simulink model "Diffsion"  (R2022b)
settings: Solver=FixedStepDiscrete  StartTime=0.0  StopTime=10.0  RelTol=1e-3
libraries: simulink x1
settings Model: Creator=yuzehong  LastModifiedBy=yuzehong
settings SolverCC: AlgebraicLoopSolver=TrustRegion
settings OptimizationCC: DefaultParameterBehavior=Inlined  EnhancedBackFolding=on  PassReuseOutputArgsAs=Individual arguments  OptimizeBlockOrder=speed  DifferentSizesBufferReuse=on  EfficientTunableParamExpr=on
settings DebuggingCC: ParameterTunabilityLossMsg=error
settings SFSimCC: MATLABDynamicMemAlloc=off
settings RTWCC: Description=Embedded Coder  SystemTargetFile=ert.tlc  GenCodeOnly=on  TemplateMakefile=ert_default_tmf
settings CodeAppCC: GenerateComments=off  IgnoreCustomStorageClasses=off  OperatorAnnotations=on  SimulinkDataObjDesc=on  SFDataObjDesc=on  SimulinkBlockComments=off
settings ERTTargetCC: TargetLangStandard=C99 (ISO)  GenerateSampleERTMain=on  CodeInterfacePackaging=Reusable function  InlinedParameterPlacement=NonHierarchical  ERTCustomFileTemplate=example_file_process.tlc

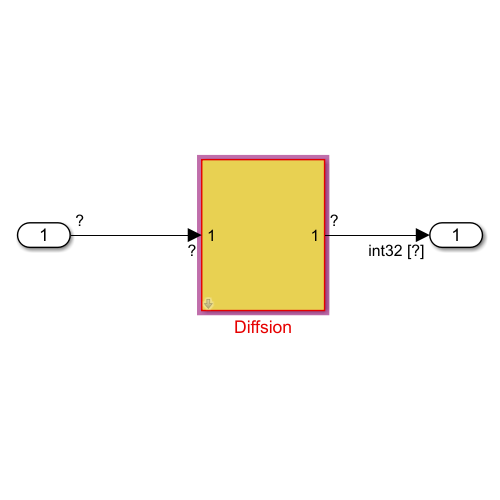
[thumbnail: Simulink's stored preview of the top-level diagram]
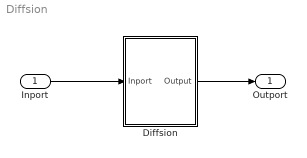
== system Diffsion ==
  Inport : Inport
  Diffsion : Subsystem  mask{length=32}
  Outport : Outport  OutDataTypeStr=int32
  wires:
  Diffsion/1(Output) -> Outport/1
  Inport/1 -> Diffsion/1(Inport)

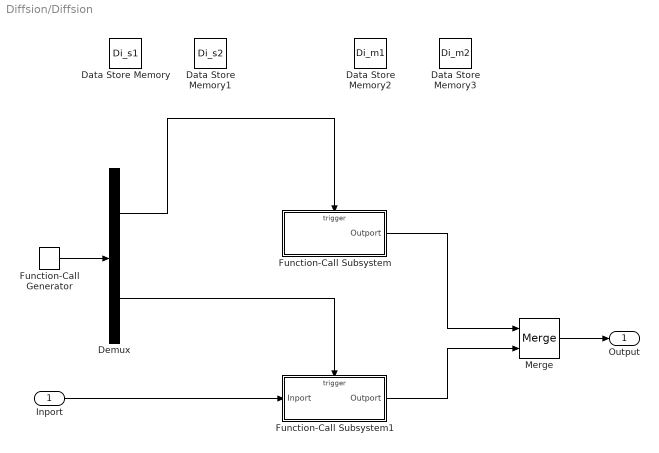
== system Diffsion/Diffsion ==
  Inport : Inport
  Data Store Memory : DataStoreMemory  DataStoreName=Di_s1  WriteAfterWriteMsg=warning  ShowAdditionalParam=off  OutDataTypeStr=int32  Dimensions=length
  Data Store Memory1 : DataStoreMemory  DataStoreName=Di_s2  WriteAfterWriteMsg=warning  ShowAdditionalParam=off  OutDataTypeStr=int32  Dimensions=length
  Data Store Memory2 : DataStoreMemory  DataStoreName=Di_m1  WriteAfterWriteMsg=warning  ShowAdditionalParam=off  OutDataTypeStr=int32  Dimensions=length
  Data Store Memory3 : DataStoreMemory  DataStoreName=Di_m2  WriteAfterWriteMsg=warning  ShowAdditionalParam=off  OutDataTypeStr=int32  Dimensions=length
  Demux : Demux  Outputs=2
  Function-Call Generator : simulink/Ports & Subsystems/Function-Call Generator  sample_time=1  numberOfIterations=1  DisallowWideOutput=off
  Function-Call Subsystem : Subsystem  TreatAsAtomicUnit=on
  Function-Call Subsystem1 : Subsystem  TreatAsAtomicUnit=on
  Merge : Merge
  Output : Outport
  wires:
  Function-Call Generator/1 -> Demux/1
  Demux/1 -> Function-Call Subsystem/Trigger
  Demux/2 -> Function-Call Subsystem1/Trigger
  Inport/1 -> Function-Call Subsystem1/1(Inport)
  Function-Call Subsystem/1(Outport) -> Merge/1
  Function-Call Subsystem1/1(Outport) -> Merge/2
  Merge/1 -> Output/1

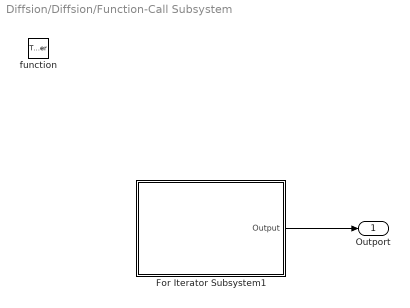
== system Diffsion/Diffsion/Function-Call Subsystem ==
  function : TriggerPort  TriggerType=function-call  VariantControl=(inherit)
  For Iterator Subsystem1 : Subsystem  TreatAsAtomicUnit=on
  Outport : Outport  OutDataTypeStr=int32
  wires:
  For Iterator Subsystem1/1(Output) -> Outport/1

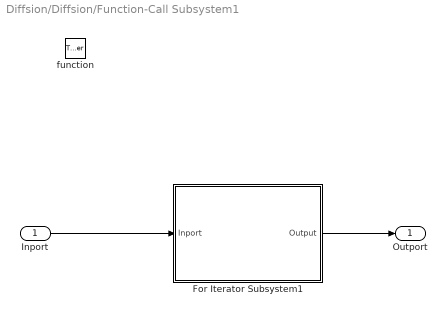
== system Diffsion/Diffsion/Function-Call Subsystem1 ==
  Inport : Inport  OutDataTypeStr=int32
  function : TriggerPort  TriggerType=function-call  VariantControl=(inherit)
  For Iterator Subsystem1 : Subsystem  TreatAsAtomicUnit=on
  Outport : Outport  OutDataTypeStr=int32
  wires:
  For Iterator Subsystem1/1(Output) -> Outport/1
  Inport/1 -> For Iterator Subsystem1/1(Inport)

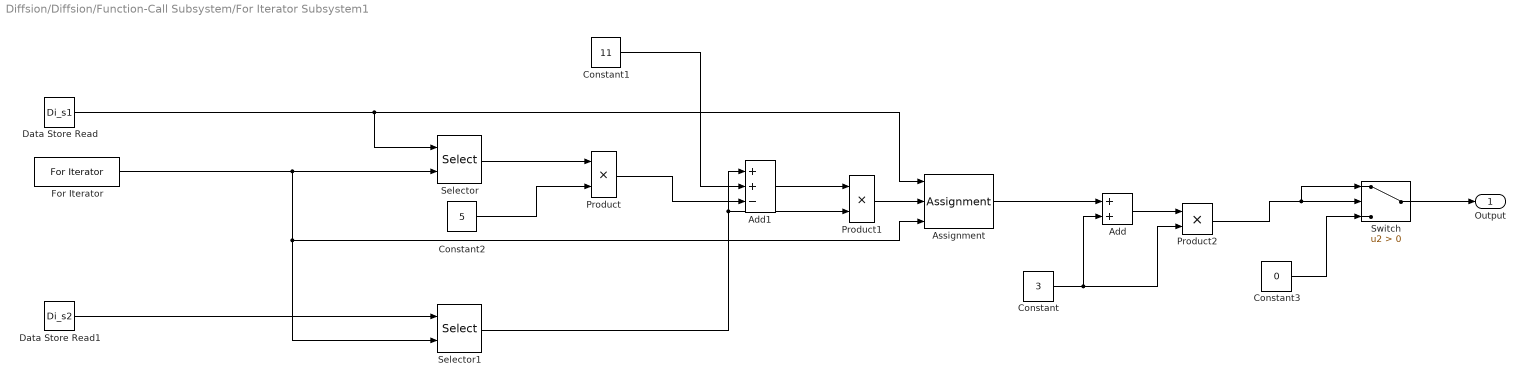
== system Diffsion/Diffsion/Function-Call Subsystem/For Iterator Subsystem1 ==
  Add : Sum  AccumDataTypeStr=int32
  Add1 : Sum  Inputs=++-  AccumDataTypeStr=int32  OutDataTypeStr=int32
  Assignment : Assignment  IndexMode=Zero-based  DiagnosticForDimensions=Warning  IndexOptions=Index vector (port)  Indices=1  OutputSizes=1
  Constant : Constant  Value=3  OutDataTypeStr=int32
  Constant1 : Constant  Value=11  OutDataTypeStr=int32
  Constant2 : Constant  Value=5  OutDataTypeStr=int32
  Constant3 : Constant  Value=0  OutDataTypeStr=int32
  Data Store Read : DataStoreRead  DataStoreName=Di_s1  IndexOptions=Index vector (dialog)  Indices=1  OutputSizes=1
  Data Store Read1 : DataStoreRead  DataStoreName=Di_s2  IndexOptions=Index vector (dialog)  Indices=1  OutputSizes=1
  For Iterator : ForIterator  IterationLimit=length  IndexMode=Zero-based
  Product : Product  OutDataTypeStr=int32
  Product1 : Product  OutDataTypeStr=int32
  Product2 : Product  OutDataTypeStr=int32
  Selector : Selector  IndexMode=Zero-based  InputPortWidth=length  IndexOptions=Index vector (port)  Indices=[1 3]  OutputSizes=1
  Selector1 : Selector  IndexMode=Zero-based  InputPortWidth=length  IndexOptions=Index vector (port)  Indices=[1 3]  OutputSizes=1
  Switch : Switch  Criteria=u2 > Threshold  SaturateOnIntegerOverflow=off  InputSameDT=off
  Output : Outport  OutDataTypeStr=int32
  wires:
  Data Store Read/1 -> Selector/1, Assignment/1
  For Iterator/1 -> Selector1/2, Assignment/3, Selector/2
  Constant2/1 -> Product/2
  Selector/1 -> Product/1
  Product/1 -> Add1/3
  Add1/1 -> Product1/1
  Product1/1 -> Assignment/2
  Constant1/1 -> Add1/2
  Data Store Read1/1 -> Selector1/1
  Selector1/1 -> Add1/1, Product1/2
  Switch/1 -> Output/1
  Constant3/1 -> Switch/3
  Assignment/1 -> Add/1
  Constant/1 -> Product2/2, Add/2
  Add/1 -> Product2/1
  Product2/1 -> Switch/1, Switch/2

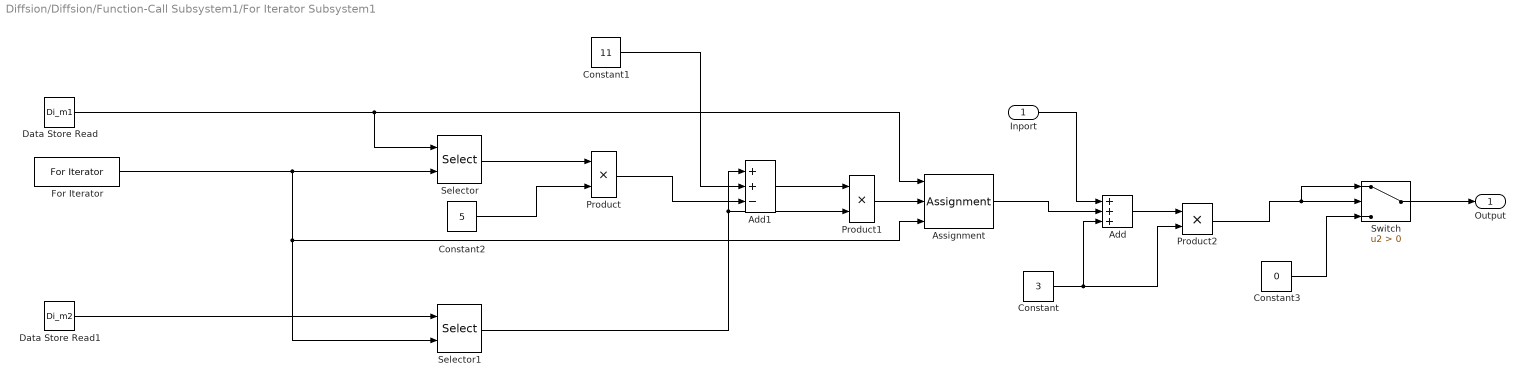
== system Diffsion/Diffsion/Function-Call Subsystem1/For Iterator Subsystem1 ==
  Inport : Inport  OutDataTypeStr=int32
  Add : Sum  Inputs=+++  AccumDataTypeStr=int32  OutDataTypeStr=int32
  Add1 : Sum  Inputs=++-  AccumDataTypeStr=int32  OutDataTypeStr=int32
  Assignment : Assignment  IndexMode=Zero-based  DiagnosticForDimensions=Warning  IndexOptions=Index vector (port)  Indices=1  OutputSizes=1
  Constant : Constant  Value=3  OutDataTypeStr=int32
  Constant1 : Constant  Value=11  OutDataTypeStr=int32
  Constant2 : Constant  Value=5  OutDataTypeStr=int32
  Constant3 : Constant  Value=0  OutDataTypeStr=int32
  Data Store Read : DataStoreRead  DataStoreName=Di_m1  IndexOptions=Index vector (dialog)  Indices=1  OutputSizes=1
  Data Store Read1 : DataStoreRead  DataStoreName=Di_m2  IndexOptions=Index vector (dialog)  Indices=1  OutputSizes=1
  For Iterator : ForIterator  IterationLimit=length  IndexMode=Zero-based
  Product : Product  OutDataTypeStr=int32
  Product1 : Product  OutDataTypeStr=int32
  Product2 : Product  OutDataTypeStr=int32
  Selector : Selector  IndexMode=Zero-based  InputPortWidth=length  IndexOptions=Index vector (port)  Indices=[1 3]  OutputSizes=1
  Selector1 : Selector  IndexMode=Zero-based  InputPortWidth=length  IndexOptions=Index vector (port)  Indices=[1 3]  OutputSizes=1
  Switch : Switch  Criteria=u2 > Threshold  SaturateOnIntegerOverflow=off  InputSameDT=off
  Output : Outport  OutDataTypeStr=int32
  wires:
  Data Store Read/1 -> Selector/1, Assignment/1
  For Iterator/1 -> Selector1/2, Assignment/3, Selector/2
  Constant2/1 -> Product/2
  Selector/1 -> Product/1
  Product/1 -> Add1/3
  Add1/1 -> Product1/1
  Product1/1 -> Assignment/2
  Constant1/1 -> Add1/2
  Data Store Read1/1 -> Selector1/1
  Selector1/1 -> Add1/1, Product1/2
  Switch/1 -> Output/1
  Constant3/1 -> Switch/3
  Assignment/1 -> Add/2
  Constant/1 -> Product2/2, Add/3
  Add/1 -> Product2/1
  Product2/1 -> Switch/1, Switch/2
  Inport/1 -> Add/1
